simulink model "quadruped_robot_jacobian"  (R2021a)
settings: Solver=ode15s  StartTime=0.0  StopTime=50  EnableMultiTasking=on
undefined symbols (not defined in the file): C, com_initial_height, H, joint_initial_q, Kvec, L, L1, L2, L3, leg1, leg2, leg3, leg4, X, Y, Z
libraries: sm_lib x52, nesl_utility x31, roblocks x8, simulink_extras x3
(part 3 of 3)

== matlab function quadruped_robot_jacobian/new_recalculate_legs_position ==
  data: u_rpy input; new_leg_pos output; legs_pos input; posCOM_W input
function new_leg_pos = new_recalculate_legs_position(u_rpy, legs_pos, posCOM_W)
% u_rpy = [roll; pitch; yaw]  (rad)
% legs_pos = [x1; y1; z1; x2; …] em frame mundo W
% posCOM_W = [x; y; z]  (centro do tronco em W)

roll  = u_rpy(1);
pitch = u_rpy(2);
yaw = u_rpy(3);

% Matriz que DESinclina
% R_nivel = rotx(rad2deg( roll )) * roty(rad2deg( pitch )); % apenas roll & pitch
R_nivel = rotx(rad2deg( roll )) * roty(rad2deg( pitch )) * rotz(rad2deg( yaw )); % roll, pitch e yaw

new_leg_pos = zeros(12,1);
for k = 1:4
    idx  = 3*(k-1)+(1:3);        % índices 1:3 4:6 …
    v_W  = legs_pos(idx) - posCOM_W;   % COM → pé
    v_B  = R_nivel \ v_W;               % remove só roll/pitch
    new_leg_pos(idx) = posCOM_W + v_B;  % alvo no mundo
end
end
